simulink model "Modello_Paolo"  (R2022b)
settings: Solver=ode113  StartTime=0.0  StopTime=t_sim  RelTol=1e-3
values from neighbouring files (symbols this model uses):
  b1 = 682.5888    [Par_Mod_Paolo.m]
  b2 = 14.6911    [Par_Mod_Paolo.m]
  cibo = 78    [Par_Mod_Paolo.m]
  cibo1 = 50    [Par_Mod_Paolo.m]
  cibo2 = 90    [Par_Mod_Paolo.m]
  cibo3 = 60    [Par_Mod_Paolo.m]
  EHP_b = 7    [Par_Mod_Paolo.m]
  G_b = 130    [Par_Mod_Paolo.m]
  G_th = 60    [Par_Mod_Paolo.m]
  h1 = 0.081389    [Par_Mod_Paolo.m]
  h3 = 0.17993    [Par_Mod_Paolo.m]
  h4 = 0.11    [Par_Mod_Paolo.m]
  h5 = 0.09    [Par_Mod_Paolo.m]
  h6 = 0.244    [Par_Mod_Paolo.m]
  H_b = 120    [Par_Mod_Paolo.m]
  I_b = 9.9345    [Par_Mod_Paolo.m]
  k = 0.10893    [Par_Mod_Paolo.m]
  k7 = 0.17079    [Par_Mod_Paolo.m]
  k8 = 0.088863    [Par_Mod_Paolo.m]
  mu = 0.00032075    [Par_Mod_Paolo.m]
  p1 = 0.0071337    [Par_Mod_Paolo.m]
  p2 = 0.046552    [Par_Mod_Paolo.m]
  p3 = 8.2334*10^(-6)    (= 8.2334e-06)    [Par_Mod_Paolo.m]
  p4 = 0.15744    [Par_Mod_Paolo.m]
  p6 = 0.031963    [Par_Mod_Paolo.m]
  p7 = 0.021764    [Par_Mod_Paolo.m]
  p8 = 0.0011994    [Par_Mod_Paolo.m]
  theta = 300    [Par_Mod_Paolo.m]
  TrePasti = 0    [Par_Mod_Paolo.m]
  Vg = 1.45    [Par_Mod_Paolo.m]
settings Model: Creator=paoga  LastModifiedBy=paoga

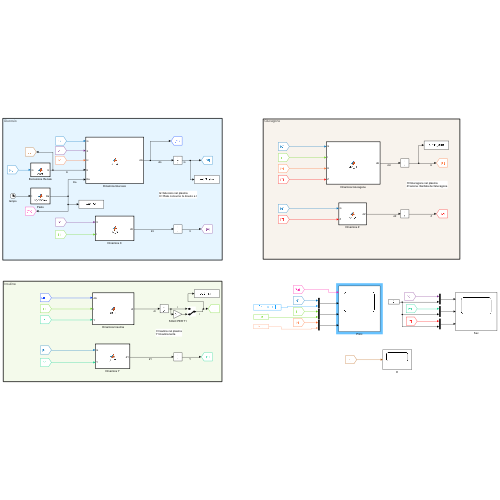
[thumbnail: Simulink's stored preview of the top-level diagram]
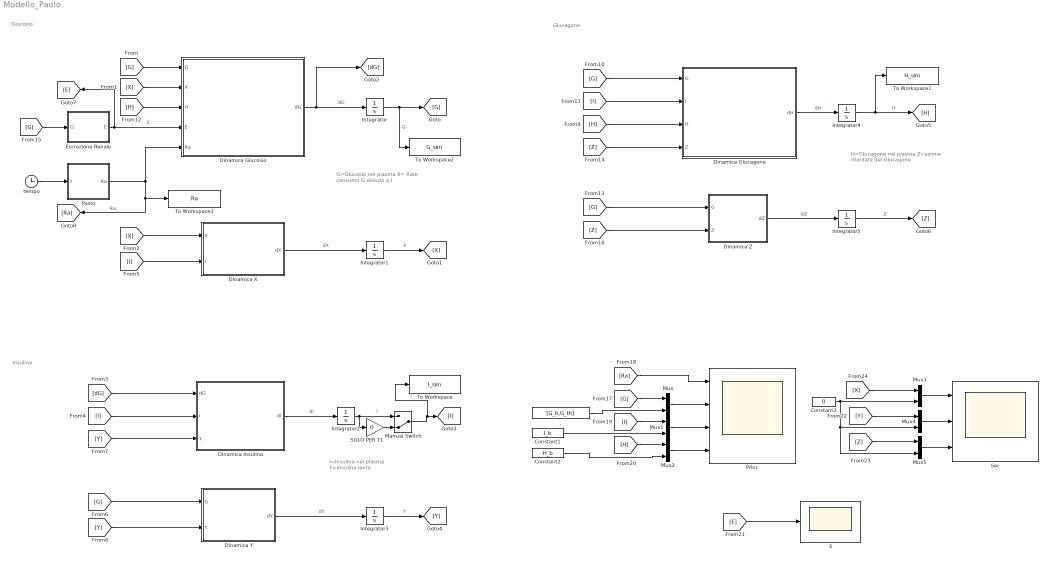
== system Modello_Paolo ==
  note: H=Glucagone nel plasma
      | Z=azione ritardata del Glucagone
  note: Glucagone
  note: I=Insulina nel plasma
      | Y=insulina lenta
  note: G=Glucosio nel plasma
      | X= Rate consumo G dovuto a I
  note: Insulina
  note: Glucosio
  "  ." : Constant  Value=[G_b,G_th]
  Constant1 : Constant  Value=I_b
  Constant2 : Constant  Value=H_b
  Constant3 : Constant  Value=0
  Dinamica Glucagone : MATLAB Function  TreatAsAtomicUnit=on
  Dinamica Glucosio : MATLAB Function  TreatAsAtomicUnit=on
  Dinamica Insulina : MATLAB Function  TreatAsAtomicUnit=on
  Dinamica X : MATLAB Function  TreatAsAtomicUnit=on
  Dinamica Y : MATLAB Function  TreatAsAtomicUnit=on
  Dinamica Z : MATLAB Function  TreatAsAtomicUnit=on
  E : Scope
  Escrezione Renale : MATLAB Function  TreatAsAtomicUnit=on
  Integrator : Integrator  InitialCondition=G_b
  Integrator1 : Integrator
  Integrator2 : Integrator  InitialCondition=I_b
  Integrator3 : Integrator
  Integrator4 : Integrator  InitialCondition=H_b
  Integrator5 : Integrator
  Manual Switch : ManualSwitch  CurrentSetting=0
  Mux{,1..5} (6 alike) : Mux  Inputs=2
  Pasto : MATLAB Function  TreatAsAtomicUnit=on
  Princ : Scope  NumInputPorts=4
  SOLO PER T1 : Gain  Gain=0
  Sec : Scope  NumInputPorts=3
  To Workspace : ToWorkspace  VariableName=I_sim  SaveFormat=Timeseries  SampleTime=-1
  To Workspace1 : ToWorkspace  VariableName=H_sim  SaveFormat=Timeseries  SampleTime=-1
  To Workspace2 : ToWorkspace  VariableName=G_sim  SaveFormat=Timeseries  SampleTime=-1
  To Workspace3 : ToWorkspace  VariableName=Ra  SaveFormat=Timeseries  SampleTime=-1
  tempo : Clock
  wires:
  Dinamica Glucosio/1(dG) -> [dG], Integrator/1  "dG"
  Integrator/1 -> To Workspace2/1, [G]  "G"
  [G] -> Dinamica Glucosio/1(G)
  Pasto/1(Ra) -> Dinamica Glucosio/5(Ra), [Ra], To Workspace3/1  "Ra"
  tempo/1 -> Pasto/1(t)
  Dinamica X/1(dX) -> Integrator1/1  "dX"
  Integrator1/1 -> [X]  "X"
  [X] -> Dinamica Glucosio/2(X)
  [X] -> Dinamica X/1(X)
  [dG] -> Dinamica Insulina/1(dG)
  Dinamica Insulina/1(dI) -> Integrator2/1  "dI"
  Integrator2/1 -> SOLO PER T1/1, Manual Switch/1  "I"
  [I] -> Dinamica Insulina/2(I)
  [I] -> Dinamica X/2(I)
  [G] -> Dinamica Y/1(G)
  Dinamica Y/1(dY) -> Integrator3/1  "dY"
  Integrator3/1 -> [Y]  "Y"
  [Y] -> Dinamica Insulina/3(Y)
  [Y] -> Dinamica Y/2(Y)
  Dinamica Glucagone/1(dH) -> Integrator4/1  "dH"
  Integrator4/1 -> To Workspace1/1, [H]  "H"
  [H] -> Dinamica Glucagone/3(H)
  [G] -> Dinamica Glucagone/1(G)
  [I] -> Dinamica Glucagone/2(I)
  [H] -> Dinamica Glucosio/3(H)
  [G] -> Dinamica Z/1(G)
  Dinamica Z/1(dZ) -> Integrator5/1  "dZ"
  Integrator5/1 -> [Z]  "Z"
  [Z] -> Dinamica Glucagone/4(Z)
  Escrezione Renale/1(E) -> Dinamica Glucosio/4(E), [E]  "E"
  [G] -> Escrezione Renale/1(G)
  [Z] -> Dinamica Z/2(Z)
  [Ra] -> Princ/1
  [G] -> Mux/1
  [I] -> Mux1/1
  [H] -> Mux2/1
  [E] -> E/1
  [X] -> Mux3/1
  [Y] -> Mux4/1
  [Z] -> Mux5/1
  "  ."/1 -> Mux/2
  Mux/1 -> Princ/2
  Mux1/1 -> Princ/3
  Constant1/1 -> Mux1/2
  Constant2/1 -> Mux2/2
  Mux2/1 -> Princ/4
  Constant3/1 -> Mux5/2, Mux4/2, Mux3/2
  Mux3/1 -> Sec/1
  Mux4/1 -> Sec/2
  Mux5/1 -> Sec/3
  SOLO PER T1/1 -> Manual Switch/2
  Manual Switch/1 -> To Workspace/1, [I]  "I"

== matlab function Modello_Paolo/Dinamica Z ==
  data: G input; dZ output; Z input; h5 parameter; h6 parameter; G_b parameter
function dZ = din_Z(G,Z,h5, h6, G_b)

if G<G_b
    dZ = -h5*Z + h6*(G_b-G);
else % se G>=G_b
    dZ=-h5*Z;
end

== matlab function Modello_Paolo/Escrezione Renale ==
  data: G input; E output; theta parameter; mu parameter
function E = escr(G,theta, mu)

if G>theta
    E = mu*(G-theta);
else
    E=0;
end

== matlab function Modello_Paolo/Pasto ==
  data: t input; Ra output; cibo parameter; b1 parameter; b2 parameter; e1 parameter; e2 parameter; TrePasti parameter; cibo1 parameter; cibo2 parameter; cibo3 parameter
function Ra = digestione(t,cibo,b1, b2, e1, e2,TrePasti, cibo1, cibo2, cibo3)

if TrePasti == 0
    Ra = cibo*b1*t^(e1)*exp(-b2*t^(e2));
else
    %===== Simulazione dei 3 pasti =====%
    if t>24*60
        t=t-24*60;
    end
    if t < 8*60 % prima di otto ore fa solo un pasto
        Ra_1 = cibo1*b1*t^(e1)*exp(-b2*t^(e2));
        Ra_2 = 0;
        Ra_3 = 0;
    elseif t >= 8*60 && t<16*60
        Ra_1 = cibo1*b1*t^(e1)*exp(-b2*t^(e2));
        Ra_2 = cibo2*b1*(t-8*60)^(e1)*exp(-b2*(t-8*60)^(e2));
        Ra_3 = 0;
    else
        Ra_1 = cibo1*b1*t^(e1)*exp(-b2*t^(e2));
        Ra_2 = cibo2*b1*(t-8*60)^(e1)*exp(-b2*(t-8*60)^(e2));
        Ra_3 = cibo3*b1*(t-16*60)^(e1)*exp(-b2*(t-16*60)^(e2));
    end

    Ra = Ra_1 + Ra_2 + Ra_3;
end

== matlab function Modello_Paolo/Dinamica Glucosio ==
  data: G input; dG output; X input; H input; E input; Ra input; p1 parameter; G_b parameter; Vg parameter; k7 parameter; k8 parameter; H_b parameter
function dG = din_G(G,X,H,E,Ra,p1, G_b, Vg, k7, k8, H_b)

dG = -(p1+X)*G + p1*G_b + Ra/Vg + ( k7*H/(k8+H) - k7*H_b/(k8+H_b) ) - E;

== matlab function Modello_Paolo/Dinamica X ==
  data: dX output; X input; I input; p2 parameter; p3 parameter; I_b parameter
function dX = din_X(X,I,p2, p3, I_b)

dX = -p2*X + p3*(I-I_b);

== matlab function Modello_Paolo/Dinamica Insulina ==
  data: dG input; I input; dI output; Y input; p4 parameter; k parameter; p6 parameter; I_b parameter
function dI = din_I(dG,I,Y,p4, k, p6, I_b)

dI = p4*Y + k*dG - p6*(I-I_b);

== matlab function Modello_Paolo/Dinamica Y ==
  data: G input; dY output; Y input; p7 parameter; p8 parameter; G_b parameter
function dY = din_Y(G,Y,p7, p8, G_b)

if G>G_b
    dY = -p7*Y + p8*(G-G_b);
else % G <= G_b
    dY = -p7*Y;
end

== matlab function Modello_Paolo/Dinamica Glucagone ==
  data: G input; I input; dH output; H input; Z input; h1 parameter; H_b parameter; EHP_b parameter; G_th parameter; h3 parameter; h4 parameter; I_b parameter; G_b parameter
function dH = din_H(G,I,H,Z, h1, H_b, EHP_b, G_th, h3, h4,I_b,G_b)

% h2=EHP_b*(h3*I_b+1)/(G_b-G_th) per rispettare la condizione di regime

dH = -h1*(H-H_b) + ( EHP_b*(h3*I_b+1)/(G_b-G_th) )*(G_th-G)/(h3*I+1) + EHP_b + h4*Z;
